simulink model "Engine_Vehicle_CVT_RS_System2"  (R2014b)
settings: Solver=ode23t  StartTime=0.0  StopTime=200  RelTol=1e-3
PostLoadFcn:
  |  load('Initialization_v2.mat');
undefined symbols (not defined in the file): sigbuilder_block, Vehicle_Mass_kg
libraries: fl_lib x16, nesl_utility x12, sdl_lib x7, simulink x4
settings Model: PauseTimes=5.041  Creator=wnursilo  LastModifiedBy=Raymond
settings SolverCC: ZeroCrossAlgorithm=Adaptive  AlgebraicLoopSolver=LineSearch
settings SimscapeCC: SimscapeLogType=all  SimscapeLogLimitData=off

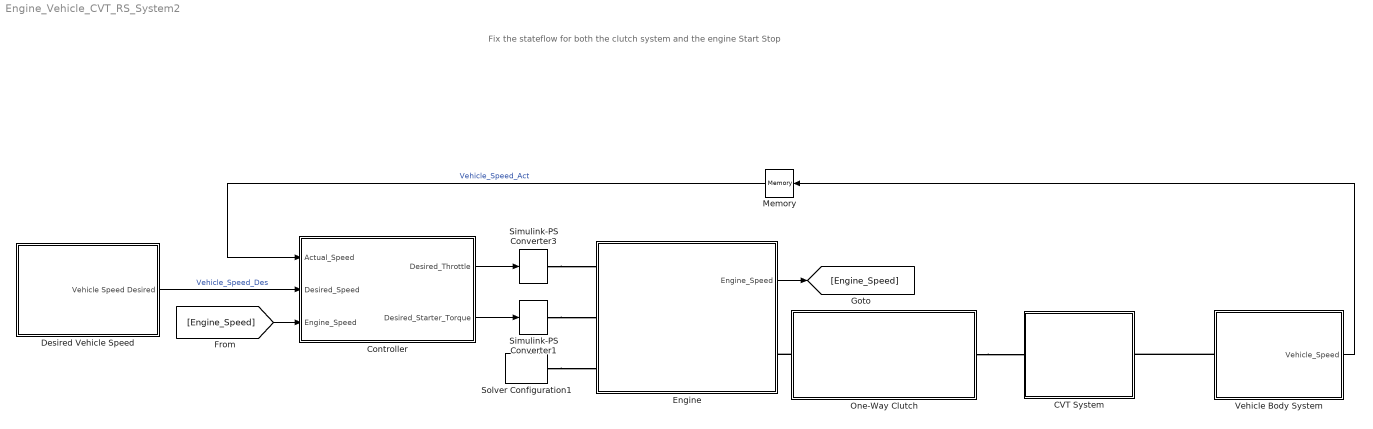
== system Engine_Vehicle_CVT_RS_System2 ==
  note: Fix the stateflow for both the clutch system and the engine Start Stop
  CVT System : Subsystem
  Controller : Subsystem
  Desired Vehicle Speed : Subsystem
  Engine : Subsystem
  Memory : Memory
  One-Way Clutch : Subsystem
  Simulink-PS Converter1 : nesl_utility/Simulink-PS Converter  PhysicalDomain=network_engine_domain  SubClassName=ps_input  LeftPortType=input  RightPortType=output  PseudoPeriodic=off  Frequencies=[]  NoiseDistribution=none  NoiseParameters=[]  Unit=N*m  AffineConversion=off  InputFiltering=on  SimscapeFilterOrder=1  InputFilterTimeConstant=0.001  UdotUserProvided=1
  Simulink-PS Converter3 : nesl_utility/Simulink-PS Converter  PhysicalDomain=network_engine_domain  SubClassName=ps_input  LeftPortType=input  RightPortType=output  PseudoPeriodic=off  Frequencies=[]  NoiseDistribution=none  NoiseParameters=[]  Unit=1  AffineConversion=off  InputFiltering=on  SimscapeFilterOrder=1  InputFilterTimeConstant=0.001  UdotUserProvided=1
  Solver Configuration1 : nesl_utility/Solver Configuration  PhysicalDomain=network_engine_domain  SubClassName=solver  LeftPortType=input  RightPortType=generic  Accelerate=off  Tones=[]  Harmonics=[]  SimulateNoise=off  Profile=off  UseLocalSampling=off  EnableSwitchedLinearOptims=on  FrequencyDomain=off  UseCCode=off  RelTol=0.001  AbsTol=1e-06  MinStep=1e-09  ToWorkspace=off  DoDC=off  ResidualTolerance=1e-09  UseLocalSolver=off  LocalSolverChoice=NE_BACKWARD_EULER_ADVANCER  LocalSolverSampleTime=0.001  DoFixedCost=off  MaxNonlinIter=3  MaxModeIter=2  LinearAlgebra=Sparse  DelaysMemoryBudget=1024  AutomaticFiltering=on  FilteringTimeConstant=0.001
  Vehicle Body System : Subsystem
  wires:
  Memory/1 -> Controller/1(Actual_Speed)  "Vehicle_Speed_Act"
  Desired Vehicle Speed/1(Vehicle Speed Desired) -> Controller/2(Desired_Speed)  "Vehicle_Speed_Des"
  Controller/1(Desired_Throttle) -> Simulink-PS Converter3/1
  Controller/2(Desired_Starter_Torque) -> Simulink-PS Converter1/1
  Vehicle Body System/1(Vehicle_Speed) -> Memory/1
  Engine/1(Engine_Speed) -> [Engine_Speed]
  [Engine_Speed] -> Controller/3(Engine_Speed)
  connections:
  Simulink-PS Converter1/RConn1 -- Engine/LConn2
  One-Way Clutch/RConn1 -- CVT System/LConn1
  One-Way Clutch/LConn1 -- Engine/RConn1
  Simulink-PS Converter3/RConn1 -- Engine/LConn1
  Vehicle Body System/LConn1 -- CVT System/RConn1
  Solver Configuration1/RConn1 -- Engine/LConn3

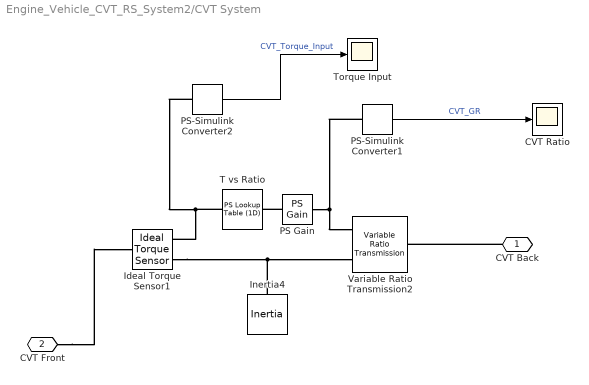
== system Engine_Vehicle_CVT_RS_System2/CVT System ==
  CVT Ratio : Scope
      settings: YMin=2  YMax=22
  Ideal Torque Sensor1 : fl_lib/Mechanical/Mechanical Sensors/Ideal Torque Sensor
  Inertia4 : fl_lib/Mechanical/Rotational Elements/Inertia  inertia=0.005 kg*m^2  w_specify=on  w_priority=High  w=0 rad/s  t_specify=off  t_priority=High  t=0 N*m
  PS Gain : fl_lib/Physical Signals/Functions/PS Gain  gain=8.5
  PS-Simulink Converter1 : nesl_utility/PS-Simulink Converter  PhysicalDomain=network_engine_domain  SubClassName=ps_output  LeftPortType=input  RightPortType=output  PseudoPeriodic=off  Frequencies=[]  Unit=1  AffineConversion=off
  PS-Simulink Converter2 : nesl_utility/PS-Simulink Converter  PhysicalDomain=network_engine_domain  SubClassName=ps_output  LeftPortType=input  RightPortType=output  PseudoPeriodic=off  Frequencies=[]  Unit=1  AffineConversion=off
  T vs Ratio : fl_lib/Physical Signals/Lookup Tables/PS Lookup Table (1D)  x_t=[9.08 0]  y_t=[1/0.4 1/2.5]  interp_method=1  extrap_method=1
  Torque Input : Scope
      settings: YMin=-2  YMax=14  SaveName=ScopeData8
  Variable Ratio Transmission2 : sdl_lib/Couplings & Drives/Variable Ratio Transmission  rotation_direction=1  kp=3e+5 N*m/rad  kv=200 N*m/(rad/s)  initial_torque=0 N*m  losses_model=1  efficiency=0.8  mu_visc=[ 0 0] N*m/(rad/s)  w_thr=0.01 rad/s
  CVT Back : PMIOPort  Port=1  Side=Right
  CVT Front : PMIOPort  Port=2  Side=Left
  wires:
  PS-Simulink Converter1/1 -> CVT Ratio/1  "CVT_GR"
  PS-Simulink Converter2/1 -> Torque Input/1  "CVT_Torque_Input"
  connections:
  CVT Back/RConn1 -- Variable Ratio Transmission2/RConn1
  PS-Simulink Converter1/LConn1 -- PS Gain/RConn1 -- Variable Ratio Transmission2/LConn1
  Ideal Torque Sensor1/RConn1 -- Inertia4/LConn1 -- Variable Ratio Transmission2/LConn2
  T vs Ratio/LConn1 -- PS-Simulink Converter2/LConn1 -- Ideal Torque Sensor1/RConn2
  PS Gain/LConn1 -- T vs Ratio/RConn1
  CVT Front/RConn1 -- Ideal Torque Sensor1/LConn1

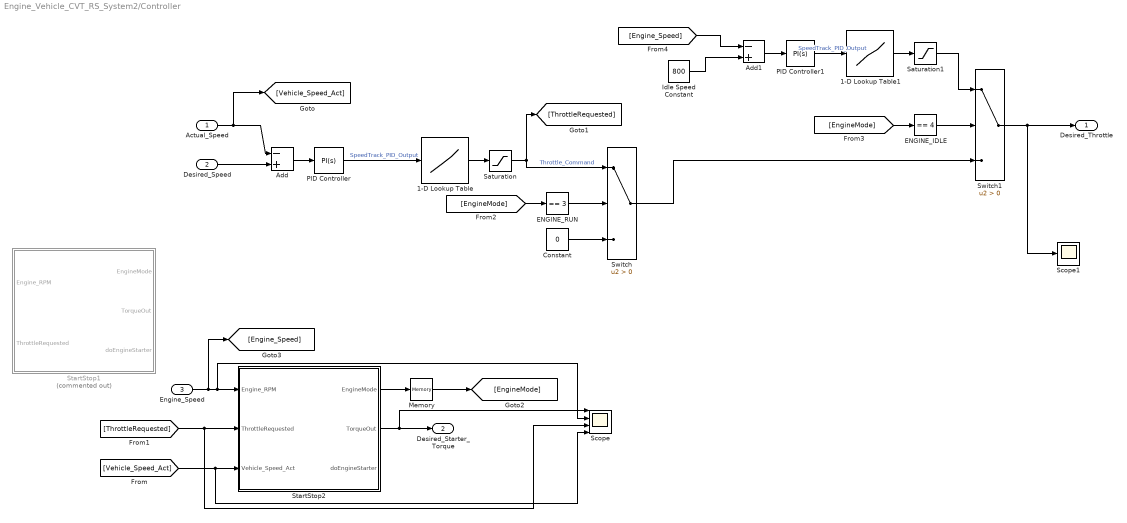
== system Engine_Vehicle_CVT_RS_System2/Controller ==
  Actual_Speed : Inport
  Desired_Speed : Inport  Port=2
  Engine_Speed : Inport  Port=3
  1-D Lookup Table : Lookup_n-D  NumberOfTableDimensions=1  BreakpointsForDimension1=[0 15]  Table=[0 1]  RndMeth=Simplest  InputSameDT=on
  1-D Lookup Table1 : Lookup_n-D  NumberOfTableDimensions=1  BreakpointsForDimension1=[0 15]  Table=[0 1]  RndMeth=Simplest  InputSameDT=on
  Add : Sum  Inputs=-+
  Add1 : Sum  Inputs=-+
  Constant : Constant  Value=0
  ENGINE_IDLE : simulink/Logic and Bit Operations/Compare To Constant  relop===  const=4  OutDataTypeStr=boolean
  ENGINE_RUN : simulink/Logic and Bit Operations/Compare To Constant  relop===  const=3  OutDataTypeStr=boolean
  Idle Speed Constant : Constant  Value=800
  Memory : Memory
  PID Controller : simulink/Continuous/PID Controller  Controller=PI  TimeDomain=Continuous-time  SampleTime=-1  IntegratorMethod=Forward Euler  FilterMethod=Forward Euler  Form=Parallel  P=2  I=0.25  D=3  N=0.1  InitialConditionSource=internal  InitialConditionForIntegrator=0  InitialConditionForFilter=0  ExternalReset=none  LimitOutput=on  UpperSaturationLimit=100  LowerSaturationLimit=0  LinearizeAsGain=on  AntiWindupMode=clamping  Kb=1  TrackingMode=off  Kt=1  PParamMin=[]  PParamMax=[]  IParamMin=[]  IParamMax=[]  DParamMin=[]  DParamMax=[]  NParamMin=[]  NParamMax=[]  KbParamMin=[]  KbParamMax=[]  KtParamMin=[]  KtParamMax=[]  POutMin=[]  POutMax=[]  IOutMin=[]  IOutMax=[]  DOutMin=[]  DOutMax=[]  NOutMin=[]  NOutMax=[]  KbOutMin=[]  KbOutMax=[]  KtOutMin=[]  KtOutMax=[]  IntegratorOutMin=[]  IntegratorOutMax=[]  FilterOutMin=[]  FilterOutMax=[]  SumOutMin=[]  SumOutMax=[]  SumI1OutMin=[]  SumI1OutMax=[]  SumI2OutMin=[]  SumI2OutMax=[]  SumI3OutMin=[]  SumI3OutMax=[]  SumDOutMin=[]  SumDOutMax=[]  SaturationOutMin=[]  SaturationOutMax=[]  IntegratorContinuousStateAttributes=''  IntegratorStateMustResolveToSignalObject=off  IntegratorRTWStateStorageClass=Auto  FilterContinuousStateAttributes=''  FilterStateMustResolveToSignalObject=off  FilterRTWStateStorageClass=Auto  DifferentiatorICPrevScaledInput=0  DifferentiatorOutMin=[]  DifferentiatorOutMax=[]  UseFilter=on
  PID Controller1 : simulink/Continuous/PID Controller  Controller=PI  TimeDomain=Continuous-time  SampleTime=-1  IntegratorMethod=Forward Euler  FilterMethod=Forward Euler  Form=Parallel  P=2  I=0.25  D=3  N=0.1  InitialConditionSource=internal  InitialConditionForIntegrator=0  InitialConditionForFilter=0  ExternalReset=none  LimitOutput=on  UpperSaturationLimit=100  LowerSaturationLimit=0  LinearizeAsGain=on  AntiWindupMode=clamping  Kb=1  TrackingMode=off  Kt=1  PParamMin=[]  PParamMax=[]  IParamMin=[]  IParamMax=[]  DParamMin=[]  DParamMax=[]  NParamMin=[]  NParamMax=[]  KbParamMin=[]  KbParamMax=[]  KtParamMin=[]  KtParamMax=[]  POutMin=[]  POutMax=[]  IOutMin=[]  IOutMax=[]  DOutMin=[]  DOutMax=[]  NOutMin=[]  NOutMax=[]  KbOutMin=[]  KbOutMax=[]  KtOutMin=[]  KtOutMax=[]  IntegratorOutMin=[]  IntegratorOutMax=[]  FilterOutMin=[]  FilterOutMax=[]  SumOutMin=[]  SumOutMax=[]  SumI1OutMin=[]  SumI1OutMax=[]  SumI2OutMin=[]  SumI2OutMax=[]  SumI3OutMin=[]  SumI3OutMax=[]  SumDOutMin=[]  SumDOutMax=[]  SaturationOutMin=[]  SaturationOutMax=[]  IntegratorContinuousStateAttributes=''  IntegratorStateMustResolveToSignalObject=off  IntegratorRTWStateStorageClass=Auto  FilterContinuousStateAttributes=''  FilterStateMustResolveToSignalObject=off  FilterRTWStateStorageClass=Auto  DifferentiatorICPrevScaledInput=0  DifferentiatorOutMin=[]  DifferentiatorOutMax=[]  UseFilter=on
  Saturation : Saturate  UpperLimit=1  LowerLimit=0
  Saturation1 : Saturate  UpperLimit=0.2  LowerLimit=0
  Scope : Scope  NumInputPorts=4
      settings: YMin=0~-200~0~-2e-31  YMax=5~800~0.8~4e-31
  Scope1 : Scope
      settings: YMin=-1  YMax=1  SaveName=ScopeData2
  StartStop1 : Stateflow chart  Commented=on  TreatAsAtomicUnit=on
  StartStop2 : Stateflow chart  TreatAsAtomicUnit=on
  Switch : Switch  Criteria=u2 > Threshold
  Switch1 : Switch  Criteria=u2 > Threshold
  Desired_Throttle : Outport
  Desired_Starter_Torque : Outport  Port=2
  wires:
  Desired_Speed/1 -> Add/2
  Add/1 -> PID Controller/1
  1-D Lookup Table/1 -> Saturation/1
  PID Controller/1 -> 1-D Lookup Table/1  "SpeedTrack_PID_Output"
  Saturation/1 -> Switch/1, [ThrottleRequested]  "Throttle_Command"
  StartStop2/2(TorqueOut) -> Scope/1, Desired_Starter_Torque/1
  Actual_Speed/1 -> [Vehicle_Speed_Act], Add/1
  Engine_Speed/1 -> [Engine_Speed], Scope/2, StartStop2/1(Engine_RPM)
  [Vehicle_Speed_Act] -> Scope/4, StartStop2/3(Vehicle_Speed_Act)
  StartStop2/1(EngineMode) -> Memory/1
  ENGINE_RUN/1 -> Switch/2
  [EngineMode] -> ENGINE_RUN/1
  Constant/1 -> Switch/3
  Switch/1 -> Switch1/3
  ENGINE_IDLE/1 -> Switch1/2
  [EngineMode] -> ENGINE_IDLE/1
  Switch1/1 -> Scope1/1, Desired_Throttle/1
  [Engine_Speed] -> Add1/1
  Idle Speed Constant/1 -> Add1/2
  Add1/1 -> PID Controller1/1
  1-D Lookup Table1/1 -> Saturation1/1
  PID Controller1/1 -> 1-D Lookup Table1/1  "SpeedTrack_PID_Output"
  Saturation1/1 -> Switch1/1
  [ThrottleRequested] -> Scope/3, StartStop2/2(ThrottleRequested)
  Memory/1 -> [EngineMode]

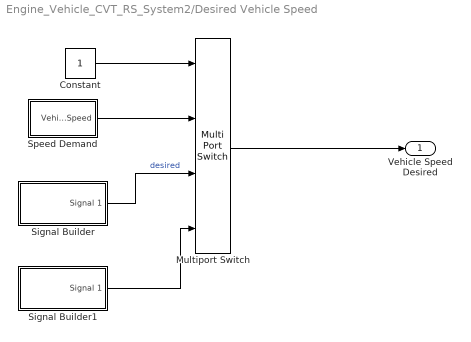
== system Engine_Vehicle_CVT_RS_System2/Desired Vehicle Speed ==
  Constant : Constant
  Multiport Switch : MultiPortSwitch
  Signal Builder : Subsystem  Tag=STV Subsys  LoadFcn=sigbuilder_block('load');  StartFcn=sigbuilder_block('start');  StopFcn=sigbuilder_block('stop');  ClipboardFcn=sigbuilder_block('clipboard');  mask(Sigbuilder block){}
      mask help: Simulink:masks:SigbuilderBlock_MD
      mask init:
      | if ~strcmp(get_param(bdroot(gcbh),'SimulationStatus'),'stopped') tuvar = sigbuilder_block('maskInit'); end
      settings: CopyFcn=sigbuilder_block('copy');  DeleteFcn=sigbuilder_block('delete');  ModelCloseFcn=sigbuilder_block('modelClose');  PreSaveFcn=sigbuilder_block('preSave');  PauseFcn=sigbuilder_block('pause');  ContinueFcn=sigbuilder_block('continue');  NameChangeFcn=sigbuilder_block('namechange');  OpenFcn=sigbuilder_block('open',[437.25 199.5 550.5 399.75 ]);  CloseFcn=sigbuilder_block('close');
      mask Display: plot(0, 0, 100, 100,[2, 2, 32, 32, 2], [68, 8, 8, 68, 68],[32, 2], [38, 38], [32, 19, 2],[53, 60, 44], [32, 17, 17, 2],[16, 16, 31, 31]);txt = getActiveGroup(gcbh);text(2, 100, txt,'verticalAlignment', 'top');
  Signal Builder1 : Subsystem  Tag=STV Subsys  LoadFcn=sigbuilder_block('load');  StartFcn=sigbuilder_block('start');  StopFcn=sigbuilder_block('stop');  ClipboardFcn=sigbuilder_block('clipboard');  mask(Sigbuilder block){}
      mask help: Simulink:masks:SigbuilderBlock_MD
      mask init:
      | if ~strcmp(get_param(bdroot(gcbh),'SimulationStatus'),'stopped') tuvar = sigbuilder_block('maskInit'); end
      settings: CopyFcn=sigbuilder_block('copy');  DeleteFcn=sigbuilder_block('delete');  ModelCloseFcn=sigbuilder_block('modelClose');  PreSaveFcn=sigbuilder_block('preSave');  PauseFcn=sigbuilder_block('pause');  ContinueFcn=sigbuilder_block('continue');  NameChangeFcn=sigbuilder_block('namechange');  OpenFcn=sigbuilder_block('open',[437.25 199.5 550.5 399.75 ]);  CloseFcn=sigbuilder_block('close');
      mask Display: plot(0, 0, 100, 100,[2, 2, 32, 32, 2], [68, 8, 8, 68, 68],[32, 2], [38, 38], [32, 19, 2],[53, 60, 44], [32, 17, 17, 2],[16, 16, 31, 31]);txt = getActiveGroup(gcbh);text(2, 100, txt,'verticalAlignment', 'top');
  Speed Demand : Subsystem
      mask Display: disp('DriveCycle')
  Vehicle Speed Desired : Outport
  wires:
  Speed Demand/1(VehicleSpeed) -> Multiport Switch/2
  Signal Builder/1(Signal 1) -> Multiport Switch/3  "desired"
  Signal Builder1/1(Signal 1) -> Multiport Switch/4
  Constant/1 -> Multiport Switch/1
  Multiport Switch/1 -> Vehicle Speed Desired/1

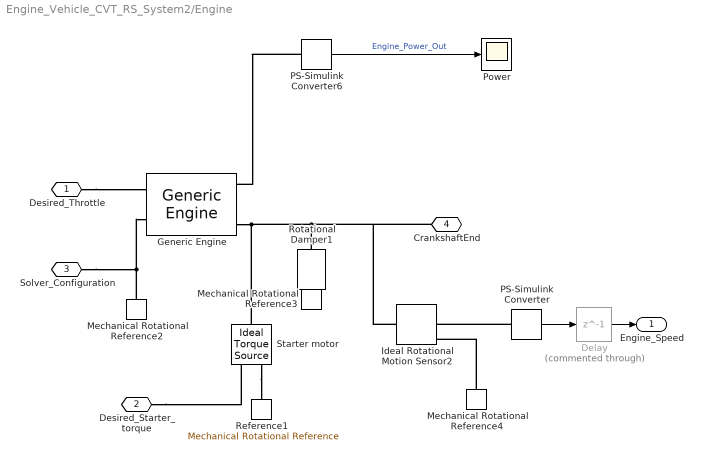
== system Engine_Vehicle_CVT_RS_System2/Engine ==
  Delay : Delay  Commented=through  DelayLength=1  InitialCondition=0  SampleTime=0.001
  Generic Engine : sdl_lib/Engines/Generic Engine  model_parameterization=1  engine_type=1  P_max=10 HP  w_P_max=8500 rpm  w_max=9000 rpm  w_min=500 rpm  w_tab=[ 500 1000 2e+3 3e+3 4e+3 5e+3 6e+3 7e+3 ] rpm  trq_tab=[ 380 380 380 380 350 280 200 80 ] N*m  pwr_tab=[ 2e+4 4e+4 7.8e+4 1.2e+5 1.45e+5 1.48e+5 1.25e+5 6e+4 ] W  interp_method=1  model_inertia=1  inertia=0.01 kg*m^2  initial_velocity=0 rpm  model_time_constant=0  time_constant=0.2 s  T0=0  w_thr=100 rpm  idle_speed=0  idle_speed_reference=800 rpm  tau_controller=0.01 s  idle_w_thr=10 rpm  fc_model=3  fc_per_rev=25 mg/rev  displaced_volume=400 cm^3  rev_per_cycle=2  fc_w_tab=[ 1000 2e+3 3e+3 4e+3 5e+3 6e+3 ] rpm  fc_trq_tab=[ 0 80 160 200 240 320 360 400 ] N*m  fc_tab=[ 0.5 0.9 1.4 1.6 1.9 2.7 3.4 4.4; 1 1.7 2.7 3.1 3.6 5 6 7.4; 1.4 2.7 4 4.8 5.6 7.5 8.5 10.5; 2 3.6 5.8 6.7 8 10.4 11.7 13.3; 2.5 4.8 7.9 9.4 10.8 14 16.2 18.6; 3.1 6 10.3 11.9 13.8 18.4 22 26.5 ] g/s  bmep_tab=[ 0 250 500 625 750 1000 1.15e+3 1.25e+3 ] kPa  bsfc_tab=[ 410 380 300 280 270 290 320 380; 410 370 290 270 260 270 285 320; 415 380 290 275 265 270 270 300; 420 390 310 290 285 280 280 285; 430 410 340 320 310 300 310 320; 450 430 370 340 330 330 350 380 ] g/hr/kW  fc_interp_method=1
  Ideal Rotational Motion Sensor2 : fl_lib/Mechanical/Mechanical Sensors/Ideal Rotational Motion Sensor  offset=0 rad
  Mechanical Rotational Reference2 : fl_lib/Mechanical/Rotational Elements/Mechanical Rotational Reference
  Mechanical Rotational Reference3 : fl_lib/Mechanical/Rotational Elements/Mechanical Rotational Reference
  Mechanical Rotational Reference4 : fl_lib/Mechanical/Rotational Elements/Mechanical Rotational Reference
  PS-Simulink Converter : nesl_utility/PS-Simulink Converter  PhysicalDomain=network_engine_domain  SubClassName=ps_output  LeftPortType=input  RightPortType=output  PseudoPeriodic=off  Frequencies=[]  Unit=rpm  AffineConversion=off
  PS-Simulink Converter6 : nesl_utility/PS-Simulink Converter  PhysicalDomain=network_engine_domain  SubClassName=ps_output  LeftPortType=input  RightPortType=output  PseudoPeriodic=off  Frequencies=[]  Unit=1  AffineConversion=off
  Power : Scope
      settings: YMin=0  YMax=7000  SaveName=ScopeData10
  Reference1 : fl_lib/Mechanical/Rotational Elements/Mechanical Rotational Reference
  Rotational Damper1 : fl_lib/Mechanical/Rotational Elements/Rotational Damper  D=0.01 N*m/(rad/s)  w_specify=off  w_priority=High  w=0 rad/s  t_specify=off  t_priority=High  t=0 N*m
  Starter motor : fl_lib/Mechanical/Mechanical Sources/Ideal Torque Source
  Desired_Throttle : PMIOPort  Port=1  Side=Left
  Desired_Starter_torque : PMIOPort  Port=2  Side=Left
  Solver_Configuration : PMIOPort  Port=3  Side=Left
  "CrankshaftEnd " : PMIOPort  Port=4  Side=Right
  Engine_Speed : Outport
  wires:
  PS-Simulink Converter6/1 -> Power/1  "Engine_Power_Out"
  PS-Simulink Converter/1 -> Delay/1
  Delay/1 -> Engine_Speed/1
  connections:
  Solver_Configuration/RConn1 -- Mechanical Rotational Reference2/LConn1 -- Generic Engine/LConn2
  Desired_Throttle/RConn1 -- Generic Engine/LConn1
  PS-Simulink Converter6/LConn1 -- Generic Engine/RConn1
  Starter motor/RConn2 -- Reference1/LConn1
  Rotational Damper1/LConn1 -- Ideal Rotational Motion Sensor2/LConn1 -- "CrankshaftEnd "/RConn1 -- Starter motor/LConn1 -- Generic Engine/RConn3
  Desired_Starter_torque/RConn1 -- Starter motor/RConn1
  Mechanical Rotational Reference3/LConn1 -- Rotational Damper1/RConn1
  PS-Simulink Converter/LConn1 -- Ideal Rotational Motion Sensor2/RConn2
  Mechanical Rotational Reference4/LConn1 -- Ideal Rotational Motion Sensor2/RConn1

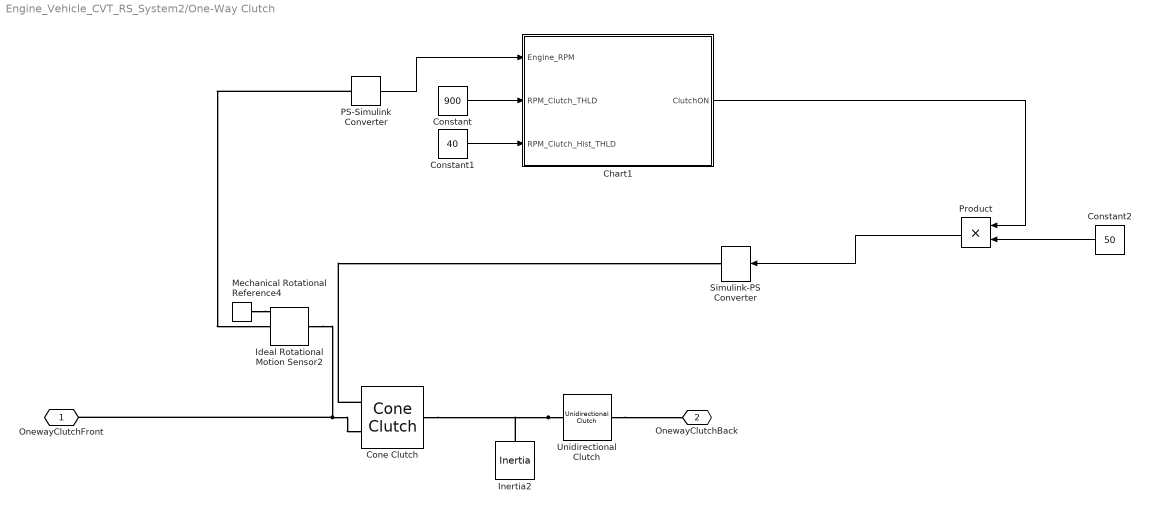
== system Engine_Vehicle_CVT_RS_System2/One-Way Clutch ==
  Chart1 : Stateflow chart  TreatAsAtomicUnit=on
  Cone Clutch : sdl_lib/Clutches/Cone Clutch  d_o=200 mm  d_i=100 mm  theta=10 deg  friction_model=1  mu_coulomb=0.25  mu_w_vector=[ 0 0.1 0.2 0.3 0.4 0.5 1 2 5 10 100 1000 ] rad/s  mu_coulomb_vector=[ 0.29 0.28 0.26 0.22 0.21 0.2 0.2 0.19 0.19 0.19 0.19 0.19 ]  mu_interp_method=1  mu_extrap_method=1  mu_static=0.5  w_tol=1 rad/s  force_min=10 N  initial_state_locked=0
  Constant : Constant  Value=900
  Constant1 : Constant  Value=40
  Constant2 : Constant  Value=50
  Ideal Rotational Motion Sensor2 : fl_lib/Mechanical/Mechanical Sensors/Ideal Rotational Motion Sensor  offset=0 rad
  Inertia2 : fl_lib/Mechanical/Rotational Elements/Inertia  inertia=0.001 kg*m^2  w_specify=on  w_priority=High  w=0 rad/s  t_specify=off  t_priority=High  t=0 N*m
  Mechanical Rotational Reference4 : fl_lib/Mechanical/Rotational Elements/Mechanical Rotational Reference
  PS-Simulink Converter : nesl_utility/PS-Simulink Converter  PhysicalDomain=network_engine_domain  SubClassName=ps_output  LeftPortType=input  RightPortType=output  PseudoPeriodic=off  Frequencies=[]  Unit=rpm  AffineConversion=off
  Product : Product
  Simulink-PS Converter : nesl_utility/Simulink-PS Converter  PhysicalDomain=network_engine_domain  SubClassName=ps_input  LeftPortType=input  RightPortType=output  PseudoPeriodic=off  Frequencies=[]  NoiseDistribution=none  NoiseParameters=[]  Unit=1  AffineConversion=off  InputFiltering=off  SimscapeFilterOrder=1  InputFilterTimeConstant=0.001  UdotUserProvided=1
  Unidirectional Clutch : sdl_lib/Clutches/Unidirectional Clutch  transmission_direction=1  initial_state_locked=0
  OnewayClutchFront : PMIOPort  Port=1  Side=Left
  OnewayClutchBack : PMIOPort  Port=2  Side=Right
  wires:
  PS-Simulink Converter/1 -> Chart1/1(Engine_RPM)
  Chart1/1(ClutchON) -> Product/1
  Constant/1 -> Chart1/2(RPM_Clutch_THLD)
  Constant1/1 -> Chart1/3(RPM_Clutch_Hist_THLD)
  Constant2/1 -> Product/2
  Product/1 -> Simulink-PS Converter/1
  connections:
  Unidirectional Clutch/RConn1 -- OnewayClutchBack/RConn1
  Unidirectional Clutch/LConn1 -- Cone Clutch/RConn1 -- Inertia2/LConn1
  Mechanical Rotational Reference4/LConn1 -- Ideal Rotational Motion Sensor2/RConn1
  Ideal Rotational Motion Sensor2/LConn1 -- Cone Clutch/LConn2 -- OnewayClutchFront/RConn1
  PS-Simulink Converter/LConn1 -- Ideal Rotational Motion Sensor2/RConn2
  Cone Clutch/LConn1 -- Simulink-PS Converter/RConn1

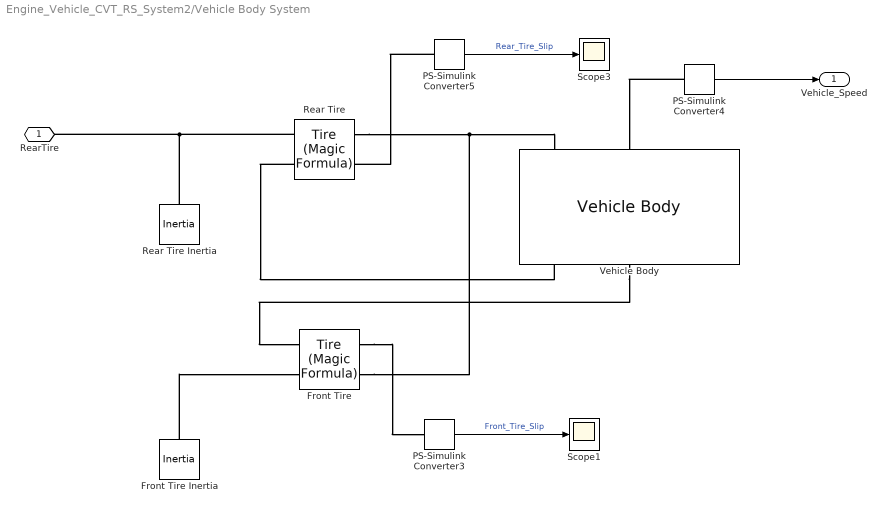
== system Engine_Vehicle_CVT_RS_System2/Vehicle Body System ==
  Front Tire Inertia : fl_lib/Mechanical/Rotational Elements/Inertia  inertia=0.01 kg*m^2  w_specify=on  w_priority=High  w=0 rad/s  t_specify=off  t_priority=High  t=0 N*m
  "Front Tire " : sdl_lib/Tires & Vehicles/Tire (Magic Formula)  parameterization=1  F_z1=Vehicle_Mass_kg*9.8/2 N  F_x1=1.5*Vehicle_Mass_kg*9.8/2 N  kappa1=10  B_m=10  C_m=1.9  D_m=1  E_m=0.97  fz0=4e+3 N  p_Cx=1.685  p_Dx=[ 1.21 -0.037 ]  p_Ex=[ 0.344 0.095 -0.02 0 ]  p_Kx=[ 21.51 -0.163 0.245 ]  p_Hx=[ -0.002 0.002 ]  p_Vx=[ 0 0 ]  v_tr_thr=0.1 m/s  r_e=0.1778 m  model_compliance=0  stiffness=1e+6 N/m  damping=1000 N/(m/s)  model_inertia=0  inertia=1 kg*m^2  initial_velocity=0 rad/s  model_resistance=0  resistance_model=1  coeff=0.015  p_tire=250e3 Pa  alpha=-0.003  beta=0.97  coeff_a=84e-4  coeff_b=6.2e-4 s/m  coeff_c=1.6e-4 s^2/m^2  v_thr=1e-3 m/s
  PS-Simulink Converter3 : nesl_utility/PS-Simulink Converter  PhysicalDomain=network_engine_domain  SubClassName=ps_output  LeftPortType=input  RightPortType=output  PseudoPeriodic=off  Frequencies=[]  Unit=1  AffineConversion=off
  PS-Simulink Converter4 : nesl_utility/PS-Simulink Converter  PhysicalDomain=network_engine_domain  SubClassName=ps_output  LeftPortType=input  RightPortType=output  PseudoPeriodic=off  Frequencies=[]  Unit=km/hr  AffineConversion=off
  PS-Simulink Converter5 : nesl_utility/PS-Simulink Converter  PhysicalDomain=network_engine_domain  SubClassName=ps_output  LeftPortType=input  RightPortType=output  PseudoPeriodic=off  Frequencies=[]  Unit=1  AffineConversion=off
  Rear Tire : sdl_lib/Tires & Vehicles/Tire (Magic Formula)  parameterization=1  F_z1=Vehicle_Mass_kg*9.8/2 N  F_x1=1.5*Vehicle_Mass_kg*9.8/2 N  kappa1=10  B_m=10  C_m=1.9  D_m=1  E_m=0.97  fz0=4e+3 N  p_Cx=1.685  p_Dx=[ 1.21 -0.037 ]  p_Ex=[ 0.344 0.095 -0.02 0 ]  p_Kx=[ 21.51 -0.163 0.245 ]  p_Hx=[ -0.002 0.002 ]  p_Vx=[ 0 0 ]  v_tr_thr=0.1 m/s  r_e=0.1778 m  model_compliance=0  stiffness=1e+6 N/m  damping=1000 N/(m/s)  model_inertia=0  inertia=1 kg*m^2  initial_velocity=0 rad/s  model_resistance=0  resistance_model=1  coeff=0.015  p_tire=250e3 Pa  alpha=-0.003  beta=0.97  coeff_a=84e-4  coeff_b=6.2e-4 s/m  coeff_c=1.6e-4 s^2/m^2  v_thr=1e-3 m/s
  Rear Tire Inertia : fl_lib/Mechanical/Rotational Elements/Inertia  inertia=0.01 kg*m^2  w_specify=on  w_priority=High  w=0 rad/s  t_specify=off  t_priority=High  t=0 N*m
  Scope1 : Scope
      settings: YMin=-3.03e-05  YMax=-3.01e-05  SaveName=ScopeData4
  Scope3 : Scope
      settings: YMin=0.0116  YMax=0.01168  SaveName=ScopeData6
  Vehicle Body : sdl_lib/Tires & Vehicles/Vehicle Body  mass=Vehicle_Mass_kg kg  n_w=1  x_f=0.75 m  x_r=0.75 m  y_c=0.5 m  area=Vehicle_FrontalArea_m2 m^2  Cd=Vehicle_DragCoef  v0=0 m/s  g=9.81 m/s^2  rho=1.18 kg/m^3
  RearTire : PMIOPort  Port=1  Side=Left
  Vehicle_Speed : Outport
  wires:
  PS-Simulink Converter3/1 -> Scope1/1  "Front_Tire_Slip"
  PS-Simulink Converter4/1 -> Vehicle_Speed/1
  PS-Simulink Converter5/1 -> Scope3/1  "Rear_Tire_Slip"
  connections:
  Rear Tire/LConn2 -- Rear Tire Inertia/LConn1 -- RearTire/RConn1
  PS-Simulink Converter4/LConn1 -- Vehicle Body/LConn2
  "Front Tire "/RConn1 -- PS-Simulink Converter3/LConn1
  PS-Simulink Converter5/LConn1 -- Rear Tire/RConn1
  Rear Tire/RConn2 -- "Front Tire "/RConn2 -- Vehicle Body/LConn1
  Rear Tire/LConn1 -- Vehicle Body/RConn1
  Front Tire Inertia/LConn1 -- "Front Tire "/LConn2
  Vehicle Body/RConn2 -- "Front Tire "/LConn1

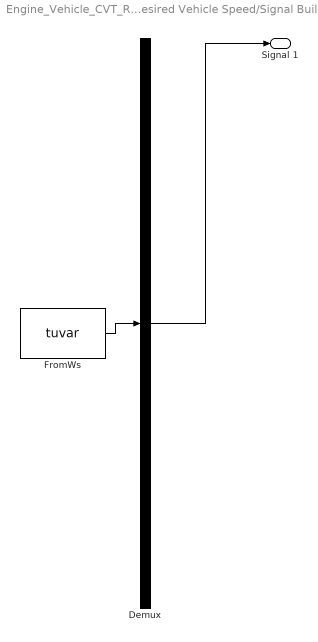
== system Engine_Vehicle_CVT_RS_System2/Desired Vehicle Speed/Signal Builder ==
  Demux : Demux  Tag=STV Demux  Outputs=1
  FromWs : FromWorkspace  Tag=STV FromWs  VariableName=tuvar  SampleTime=0
      SigBuilderData=|
      | common.afterFinalStr = 'Extrapolate'
      | common.sampleTime = 0
      | dataSet.timeRange = [0 100]
      | dataSet.name = 'Group 1'
      | sbobj.Groups.Name = 'Group 1'
      | sbobj.Groups.Signals.Name = 'Signal 1'
      | sbobj.Groups.Signals.XData = [0 5 10 20 30 35 40 45 80 90 100]
      | sbobj.Groups.Signals.YData = [0 0 60 60 52 40 40 50 45 0 0]
      | sbobj.Groups.TimeRange = [0 100]
  Signal 1 : Outport  Tag=STV Outport
  wires:
  FromWs/1 -> Demux/1
  Demux/1 -> Signal 1/1

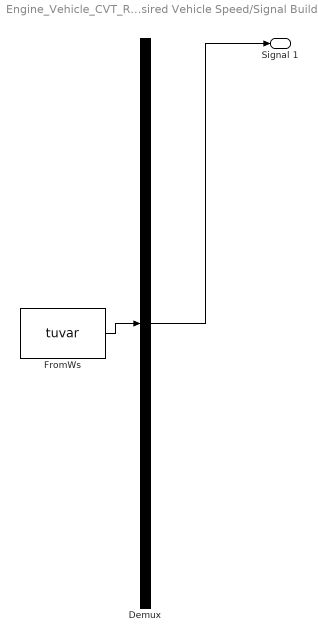
== system Engine_Vehicle_CVT_RS_System2/Desired Vehicle Speed/Signal Builder1 ==
  Demux : Demux  Tag=STV Demux  Outputs=1
  FromWs : FromWorkspace  Tag=STV FromWs  VariableName=tuvar  SampleTime=0
      SigBuilderData=|
      | common.afterFinalStr = 'Extrapolate'
      | common.sampleTime = 0
      | dataSet.timeRange = [0 100]
      | dataSet.name = 'Group 1'
      | sbobj.Groups.Name = 'Group 1'
      | sbobj.Groups.Signals.Name = 'Signal 1'
      | sbobj.Groups.Signals.XData = [0 5 10 20 30 35 40 45 60 60 65 65 80 90 100]
      | sbobj.Groups.Signals.YData = [0 0 60 60 52 0.5 0.5 50 45 0 0 21 45 0 0]
      | sbobj.Groups.TimeRange = [0 100]
  Signal 1 : Outport  Tag=STV Outport
  wires:
  Demux/1 -> Signal 1/1
  FromWs/1 -> Demux/1

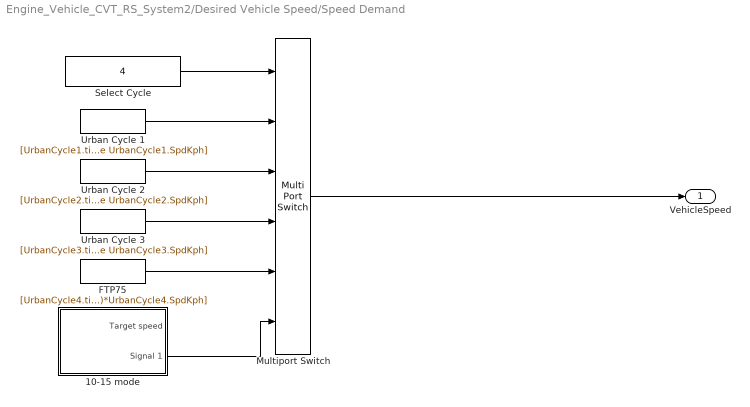
== system Engine_Vehicle_CVT_RS_System2/Desired Vehicle Speed/Speed Demand ==
  "10-15 mode " : Subsystem  Tag=STV Subsys  LoadFcn=sigbuilder_block('load');  StartFcn=sigbuilder_block('start');  StopFcn=sigbuilder_block('stop');  ClipboardFcn=sigbuilder_block('clipboard');  mask(Sigbuilder block){}
      mask help: Sigbuilder GUI
      mask init:
      | if ~strcmp(get_param(bdroot(gcbh),'SimulationStatus'),'stopped') tuvar = sigbuilder_block('maskInit'); end
      settings: CopyFcn=sigbuilder_block('copy');  DeleteFcn=sigbuilder_block('delete');  ModelCloseFcn=sigbuilder_block('modelClose');  PreSaveFcn=sigbuilder_block('preSave');  PauseFcn=sigbuilder_block('pause')  ContinueFcn=sigbuilder_block('continue')  NameChangeFcn=sigbuilder_block('namechange');  OpenFcn=sigbuilder_block('open',[5.58621 35.3793 980.69 465.517 ]);  CloseFcn=sigbuilder_block('close');
      mask Display: plot(0,0,100,100,[10,10,40,40,10],[80,20,20,80,80],[40,10],[50,50], [40,27,10],[65,72,56],[40,25,25,10],[28,28,43,43]);
  FTP75 : FromWorkspace  VariableName=[UrbanCycle4.time Vehicle_MaxSpeed_kph/max(UrbanCycle4.SpdKph)*UrbanCycle4.SpdKph]  SampleTime=0
  Multiport Switch : MultiPortSwitch  Inputs=5
  Select Cycle : Constant  Value=4
  Urban Cycle 1 : FromWorkspace  VariableName=[UrbanCycle1.time UrbanCycle1.SpdKph]  SampleTime=0
  Urban Cycle 2 : FromWorkspace  VariableName=[UrbanCycle2.time UrbanCycle2.SpdKph]  SampleTime=0
  Urban Cycle 3 : FromWorkspace  VariableName=[UrbanCycle3.time UrbanCycle3.SpdKph]  SampleTime=0
  VehicleSpeed : Outport
  wires:
  Urban Cycle 3/1 -> Multiport Switch/4
  Select Cycle/1 -> Multiport Switch/1
  Urban Cycle 2/1 -> Multiport Switch/3
  Urban Cycle 1/1 -> Multiport Switch/2
  FTP75/1 -> Multiport Switch/5
  "10-15 mode "/2(Signal 1) -> Multiport Switch/6
  Multiport Switch/1 -> VehicleSpeed/1

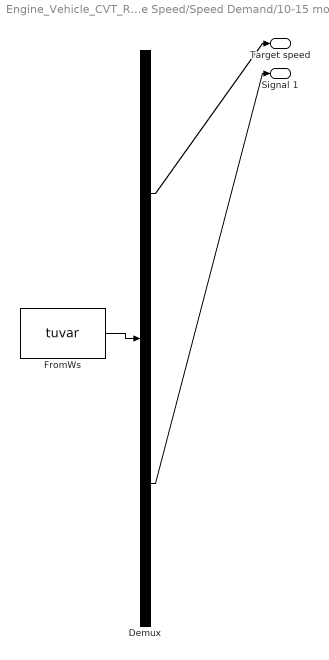
== system Engine_Vehicle_CVT_RS_System2/Desired Vehicle Speed/Speed Demand/10-15 mode  ==
  Demux : Demux  Tag=STV Demux  Outputs=2
  FromWs : FromWorkspace  Tag=STV FromWs  VariableName=tuvar  SampleTime=0
      SigBuilderData=|
      | common.afterFinalStr = 'Extrapolate'
      | common.sampleTime = '0'
      | dataSet.timeRange = [0 660]
      | dataSet.name = '10-15 Mode Cycle'
      | sbobj.Groups.Name = '10-15 Mode Cycle'
      | sbobj.Groups.Signals(1).Name = 'Target speed'
      | sbobj.Groups.Signals(1).XData = [0 44 51 73 73 89 103 118 128 130 142 152 159 179 186 201 208 224 238 253 263 265 277 287 294 314 321 336 343 359 373 388 398 400 412 422 429 494 512 524 528 532 548 558 569 579 589 593 615 620 640 650 660]
      | sbobj.Groups.Signals(1).YData = [0 0 10 10 0 0 40 40 20 20 40 20 0 0 20 20 0 0 40 40 20 20 40 20 0 0 20 20 0 0 40 40 20 20 40 20 0 0 50 50 40 40 60 60 70 70 50 50 70 70 30 0 0]
      | sbobj.Groups.Signals(2).Name = 'Signal 1'
      | sbobj.Groups.Signals(2).XData = [0 20 120 120 220 220 320 320 420 420 520 520 620 650 660]
      | sbobj.Groups.Signals(2).YData = [0 10 10 20 20 30 30 40 39.8 50 50 60 60 0.5 0]
  Target speed : Outport  Tag=STV Outport
  Signal 1 : Outport  Tag=STV Outport  Port=2
  wires:
  FromWs/1 -> Demux/1
  Demux/1 -> Target speed/1
  Demux/2 -> Signal 1/1

== stateflow chart Engine_Vehicle_CVT_RS_System2/One-Way Clutch/Chart1 ==
  (default) -> (junction 2)
  (junction 2) -> (junction 5) [order 2] : [ Engine_RPM > RPM_Clutch_THLD]
  (junction 5) -> (junction 7) : {
      | ClutchON = 1;
      | }
  (junction 2) -> (junction 3) [order 1] : [Engine_RPM < RPM_Clutch_THLD - RPM_Clutch_Hist_THLD]
      | {
      | ClutchON = 0;
      | }
  (junction 7) -> (junction 3)
  data: Engine_RPM input; RPM_Clutch_THLD input; RPM_Clutch_Hist_THLD input; ClutchON output

== stateflow chart Engine_Vehicle_CVT_RS_System2/Controller/StartStop2 ==
  state ENGINE_STOP
    entry:
    EngineMode  = STOP;
  state ENGINE_StartRequest
    entry:
    EngineMode = STARTREQUESTED;
    during:
    if before(1,sec)
    doEngineStarter = 1;
    TorqueOut = 5;
    else
    doEngineStarter = 0;
    TorqueOut = 0;
    end
  state ENGINE_IDLE
    entry:
    EngineMode  = IDLE;
  state ENGINE_Run
    entry:
    EngineMode = RUN;
    doEngineStarter = 0;
    TorqueOut = 0;
  (default) -> ENGINE_STOP
  ENGINE_IDLE -> ENGINE_STOP [order 2] : [ThrottleRequested < 0.1 && ...
      | Vehicle_Speed_Act <3]
  ENGINE_StartRequest -> ENGINE_STOP [order 1] : [Engine_RPM <800 && ...
      | doEngineStarter ==0 &&...
      | after(5,sec)]
  ENGINE_STOP -> ENGINE_StartRequest : [Engine_RPM < 800 && ...
      | ThrottleRequested > 0.1 &&...
      | after(0.2,sec)]
  ENGINE_StartRequest -> ENGINE_IDLE [order 2] : [Engine_RPM>800 &&...
      | after(0.25,sec)]
  ENGINE_IDLE -> ENGINE_Run [order 1] : [Engine_RPM > 800 &&...
      | ThrottleRequested > 0.1 && ...
      | after(0.2,sec)]
  ENGINE_Run -> ENGINE_IDLE : [ThrottleRequested <0.1 &&...
      | Vehicle_Speed_Act >= 3]
  data: EngineMode output; TorqueOut output; Engine_RPM input; ThrottleRequested input; doEngineStarter output; STARTREQUESTED constant double =2; RUN constant double =3; STOP constant double =1; Vehicle_Speed_Act input; IDLE constant double =4

== stateflow chart Engine_Vehicle_CVT_RS_System2/Controller/StartStop1 ==
  state ENGINE_STOP
    entry:
    EngineMode  = STOP;
  state ENGINE_StartRequest
    entry:
    EngineMode = StartRequest;
    during:
    if before(1,sec)
    doEngineStarter = 1;
    TorqueOut = 5;
    else
    doEngineStarter = 0;
    TorqueOut = 0;
    end
  state ENGINE_Run
    entry:
    EngineMode = Run;
    doEngineStarter = 0;
    TorqueOut = 0;
  (default) -> ENGINE_STOP
  ENGINE_Run -> ENGINE_STOP : [ThrottleRequested< 0.1 && ...
      | Engine_RPM < 800]
  ENGINE_StartRequest -> ENGINE_STOP [order 2] : [Engine_RPM <800 && ...
      | doEngineStarter ==0 &&...
      | after(5,sec)]
  ENGINE_StartRequest -> ENGINE_STOP [commented out] : [Engine_RPM <800 && ...
      | doEngineStarter ==0 &&...
      | TimeDiff > 5]
  ENGINE_STOP -> ENGINE_StartRequest : [Engine_RPM < 800 && ...
      | ThrottleRequested > 0.1 &&...
      | after(2,sec)]
  ENGINE_StartRequest -> ENGINE_Run [order 1] : [Engine_RPM > 800]
  data: EngineMode output; TorqueOut output; Engine_RPM input; ThrottleRequested input; doEngineStarter output; StartRequest constant double =2; Run constant double =3; STOP constant double =1
